simulink model "fonction"  (R2021a)
settings: Solver=VariableStepAuto  StartTime=0.0  StopTime=10.0  RelTol=1e-3
settings Model: Creator=ialouane  LastModifiedBy=ialouane

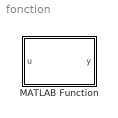
== system fonction ==
  MATLAB Function : MATLAB Function  TreatAsAtomicUnit=on

== matlab function fonction/MATLAB Function ==
  data: u input; y output
function y = fcn(u)

y = [u(2) 10*sin(u(1));
end
